simulink model "processor_128_channel_test"  (R2016b)
settings: Solver=VariableStepAuto  StartTime=0.0  StopTime=2^16/Fadc  RelTol=1e-3  EnableMultiTasking=on
PreLoadFcn:
  | setup
values from neighbouring files (symbols this model uses):
  Fadc = 614.4e6    (= 614400000)    [setup.m]
undefined symbols (not defined in the file or in its folder): etaTable, freqTable, gcbh, xlBlockLoadCallback
libraries: xbsIndex_r4 x44, CryoDetLibCMB x23, simulink x1
settings Model: Creator=Mitch  LastModifiedBy=mdewart
settings OptimizationCC: LifeSpan=inf
settings DebuggingCC: SFUnexpectedBacktrackingDiag=warning  SFNoUnconditionalDefaultTransitionDiag=warning  SFExecutionAtInitializationDiag=none
settings GRTTargetCC: TargetLangStandard=C89/C90 (ANSI)  GeneratePreprocessorConditionals=Disable all
settings ConfigComp: CovMetricSettings=dw  CovHtmlReporting=on  CovSaveCumulativeToWorkspaceVar=on  CovSaveSingleToWorkspaceVar=on  CovExternalEMLEnable=off

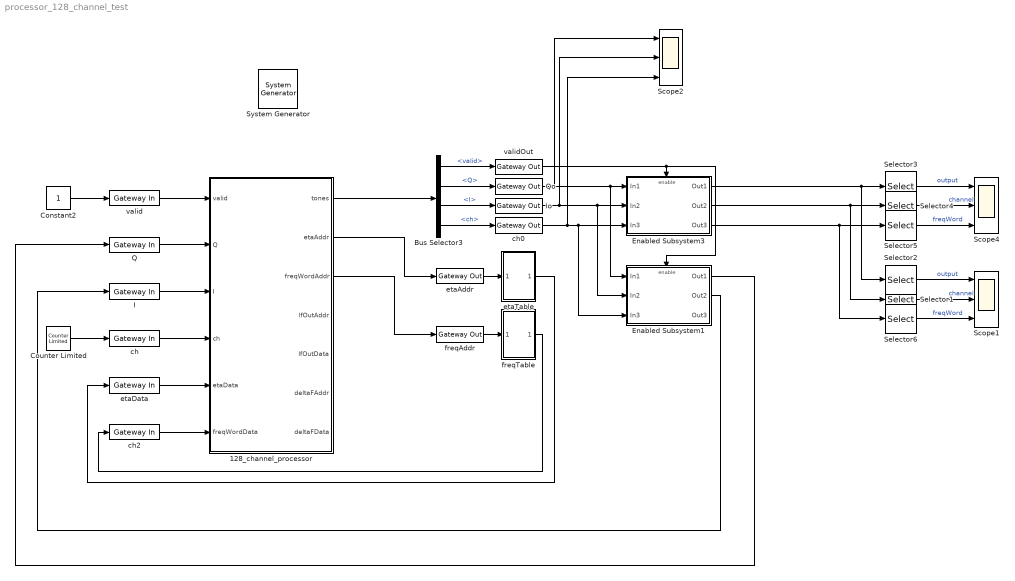
== system processor_128_channel_test ==
  " System Generator" : xbsIndex_r4/ System Generator  Tag=genX  xilinxfamily=kintexu  part=xcku040  speed=-2-e  package=ffva1156  synthesis_tool=Vivado  clock_wrapper=Clock Enables  directory=./netlist  proj_type=Vivado  Synth_file=Vivado Synthesis Defaults  Impl_file=Vivado Implementation Defaults  testbench=off  simulink_period=2/Fadc  sysclk_period=2e9/Fadc  dcm_input_clock_period=10  incr_netlist=off  trim_vbits=Everywhere in SubSystem  dbl_ovrd=According to Block Masks  core_generation=According to Block Masks  run_coregen=off  deprecated_control=off  eval_field=0  block_type=sysgen
  128_channel_processor : Subsystem  AncestorBlock=CryoDetLibCMB/128_channel_processor
  Bus Selector3 : BusSelector  OutputSignals=valid,Q,I,ch
  Constant2 : Constant  SampleTime=2/Fadc
  Counter Limited : simulink/Sources/Counter Limited  uplimit=7  tsamp=2/Fadc
  Enabled Subsystem1 : Subsystem  TreatAsAtomicUnit=on
  Enabled Subsystem3 : Subsystem  TreatAsAtomicUnit=on
  I : xbsIndex_r4/Gateway In  gui_display_data_type=Fixed-point  arith_type="Signed  (2's comp)"  n_bits=18  bin_pt=16  preci_type=Single  exp_width=8  frac_width=24  rows=1  columns=1  quantization="Round  (unbiased: +/- Inf)"  overflow=Saturate  period=2/Fadc  UseAsADC=off  ADCChannel='1'  interface=None  automatic_assignment=on  address_offset=hex2dec('00')  intf_name=''  intf_description=''  default_value=0  timing_constraint=None  locs_specified=off  LOCs={}  io_standard={}  inherit_from_input=off  hdl_port=on  dbl_ovrd=off  block_type=gatewayin
  Io : xbsIndex_r4/Gateway Out  inherit_from_input=off  hdl_port=on  rows=1  columns=1  UseAsDAC=off  DACChannel='1'  interface=None  automatic_assignment=on  address_offset=hex2dec('00')  intf_name=''  intf_description=''  timing_constraint=None  locs_specified=off  LOCs={}  io_standard={}  block_type=gatewayout
  Q : xbsIndex_r4/Gateway In  gui_display_data_type=Fixed-point  arith_type="Signed  (2's comp)"  n_bits=18  bin_pt=16  preci_type=Single  exp_width=8  frac_width=24  rows=1  columns=1  quantization="Round  (unbiased: +/- Inf)"  overflow=Saturate  period=2/Fadc  UseAsADC=off  ADCChannel='1'  interface=None  automatic_assignment=on  address_offset=hex2dec('00')  intf_name=''  intf_description=''  default_value=0  timing_constraint=None  locs_specified=off  LOCs={}  io_standard={}  inherit_from_input=off  hdl_port=on  dbl_ovrd=off  block_type=gatewayin
  Qo : xbsIndex_r4/Gateway Out  inherit_from_input=off  hdl_port=on  rows=1  columns=1  UseAsDAC=off  DACChannel='1'  interface=None  automatic_assignment=on  address_offset=hex2dec('00')  intf_name=''  intf_description=''  timing_constraint=None  locs_specified=off  LOCs={}  io_standard={}  block_type=gatewayout
  Scope1 : Scope  NumInputPorts=3
  Scope2 : Scope  NumInputPorts=3
  Scope4 : Scope  NumInputPorts=3
  Selector1 : Selector  InputPortWidth=8  IndexOptions=Index vector (dialog)  Indices=[7+1]  OutputSizes=1
  Selector2 : Selector  InputPortWidth=8  IndexOptions=Index vector (dialog)  Indices=[7+1]  OutputSizes=1
  Selector3 : Selector  InputPortWidth=8  IndexOptions=Index vector (dialog)  Indices=[1]  OutputSizes=1
  Selector4 : Selector  InputPortWidth=8  IndexOptions=Index vector (dialog)  Indices=[1]  OutputSizes=1
  Selector5 : Selector  InputPortWidth=8  IndexOptions=Index vector (dialog)  Indices=[1]  OutputSizes=1
  Selector6 : Selector  InputPortWidth=8  IndexOptions=Index vector (dialog)  Indices=[7+1]  OutputSizes=1
  ch : xbsIndex_r4/Gateway In  gui_display_data_type=Fixed-point  arith_type=Unsigned  n_bits=3  bin_pt=0  preci_type=Single  exp_width=8  frac_width=24  rows=1  columns=1  quantization="Round  (unbiased: +/- Inf)"  overflow=Saturate  period=2/Fadc  UseAsADC=off  ADCChannel='1'  interface=None  automatic_assignment=on  address_offset=hex2dec('00')  intf_name=''  intf_description=''  default_value=0  timing_constraint=None  locs_specified=off  LOCs={}  io_standard={}  inherit_from_input=off  hdl_port=on  dbl_ovrd=off  block_type=gatewayin
  ch0 : xbsIndex_r4/Gateway Out  inherit_from_input=off  hdl_port=on  rows=1  columns=1  UseAsDAC=off  DACChannel='1'  interface=None  automatic_assignment=on  address_offset=hex2dec('00')  intf_name=''  intf_description=''  timing_constraint=None  locs_specified=off  LOCs={}  io_standard={}  block_type=gatewayout
  ch2 : xbsIndex_r4/Gateway In  gui_display_data_type=Fixed-point  arith_type=Unsigned  n_bits=32  bin_pt=0  preci_type=Single  exp_width=8  frac_width=24  rows=1  columns=1  quantization="Round  (unbiased: +/- Inf)"  overflow=Saturate  period=2/Fadc  UseAsADC=off  ADCChannel='1'  interface=None  automatic_assignment=on  address_offset=hex2dec('00')  intf_name=''  intf_description=''  default_value=0  timing_constraint=None  locs_specified=off  LOCs={}  io_standard={}  inherit_from_input=off  hdl_port=on  dbl_ovrd=off  block_type=gatewayin
  etaAddr : xbsIndex_r4/Gateway Out  inherit_from_input=on  hdl_port=on  rows=1  columns=1  UseAsDAC=off  DACChannel='1'  interface=None  automatic_assignment=on  address_offset=hex2dec('00')  intf_name=''  intf_description=''  timing_constraint=None  locs_specified=off  LOCs={}  io_standard={}  block_type=gatewayout
  etaData : xbsIndex_r4/Gateway In  gui_display_data_type=Fixed-point  arith_type=Unsigned  n_bits=32  bin_pt=0  preci_type=Single  exp_width=8  frac_width=24  rows=1  columns=1  quantization="Round  (unbiased: +/- Inf)"  overflow=Saturate  period=2/Fadc  UseAsADC=off  ADCChannel='1'  interface=None  automatic_assignment=on  address_offset=hex2dec('00')  intf_name=''  intf_description=''  default_value=0  timing_constraint=None  locs_specified=off  LOCs={}  io_standard={}  inherit_from_input=off  hdl_port=on  dbl_ovrd=off  block_type=gatewayin
  etaTable : Subsystem
  freqAddr : xbsIndex_r4/Gateway Out  inherit_from_input=on  hdl_port=on  rows=1  columns=1  UseAsDAC=off  DACChannel='1'  interface=None  automatic_assignment=on  address_offset=hex2dec('00')  intf_name=''  intf_description=''  timing_constraint=None  locs_specified=off  LOCs={}  io_standard={}  block_type=gatewayout
  freqTable : Subsystem
  valid : xbsIndex_r4/Gateway In  gui_display_data_type=Boolean  arith_type=Boolean  n_bits=18  bin_pt=15  preci_type=Single  exp_width=8  frac_width=24  rows=1  columns=1  quantization="Round  (unbiased: +/- Inf)"  overflow=Saturate  period=2/Fadc  UseAsADC=off  ADCChannel='1'  interface=None  automatic_assignment=on  address_offset=hex2dec('00')  intf_name=''  intf_description=''  default_value=0  timing_constraint=None  locs_specified=off  LOCs={}  io_standard={}  inherit_from_input=off  hdl_port=on  dbl_ovrd=off  block_type=gatewayin
  validOut : xbsIndex_r4/Gateway Out  inherit_from_input=off  hdl_port=on  rows=1  columns=1  UseAsDAC=off  DACChannel='1'  interface=None  automatic_assignment=on  address_offset=hex2dec('00')  intf_name=''  intf_description=''  timing_constraint=None  locs_specified=off  LOCs={}  io_standard={}  block_type=gatewayout
  wires:
  Constant2/1 -> valid/1
  ch/1 -> 128_channel_processor/4(ch)
  valid/1 -> 128_channel_processor/1(valid)
  Bus Selector3/2 -> Qo/1  "<Q>"
  Bus Selector3/3 -> Io/1  "<I>"
  Bus Selector3/1 -> validOut/1  "<valid>"
  Bus Selector3/4 -> ch0/1  "<ch>"
  Selector3/1 -> Scope4/1  "output"
  Selector5/1 -> Scope4/3  "freqWord"
  Selector4/1 -> Scope4/2  "channel"
  Selector2/1 -> Scope1/1  "output"
  Selector6/1 -> Scope1/3  "freqWord"
  Selector1/1 -> Scope1/2  "channel"
  Q/1 -> 128_channel_processor/2(Q)
  Counter Limited/1 -> ch/1
  etaData/1 -> 128_channel_processor/5(etaData)
  ch2/1 -> 128_channel_processor/6(freqWordData)
  128_channel_processor/1(tones) -> Bus Selector3/1
  validOut/1 -> Enabled Subsystem1/Enable, Enabled Subsystem3/Enable
  ch0/1 -> Scope2/3, Enabled Subsystem1/3(In3), Enabled Subsystem3/3(In3)
  Io/1 -> Scope2/2, Enabled Subsystem1/2(In2), Enabled Subsystem3/2(In2)
  I/1 -> 128_channel_processor/3(I)
  Enabled Subsystem3/2(Out2) -> Selector1/1, Selector4/1
  128_channel_processor/2(etaAddr) -> etaAddr/1
  128_channel_processor/3(freqWordAddr) -> freqAddr/1
  Enabled Subsystem3/3(Out3) -> Selector6/1, Selector5/1
  Enabled Subsystem3/1(Out1) -> Selector2/1, Selector3/1
  etaAddr/1 -> etaTable/1(In1)
  freqAddr/1 -> freqTable/1(In1)
  freqTable/1(Out1) -> ch2/1
  etaTable/1(Out1) -> etaData/1
  Qo/1 -> Scope2/1, Enabled Subsystem1/1(In1), Enabled Subsystem3/1(In1)
  Enabled Subsystem1/1(Out1) -> Q/1
  Enabled Subsystem1/2(Out2) -> I/1

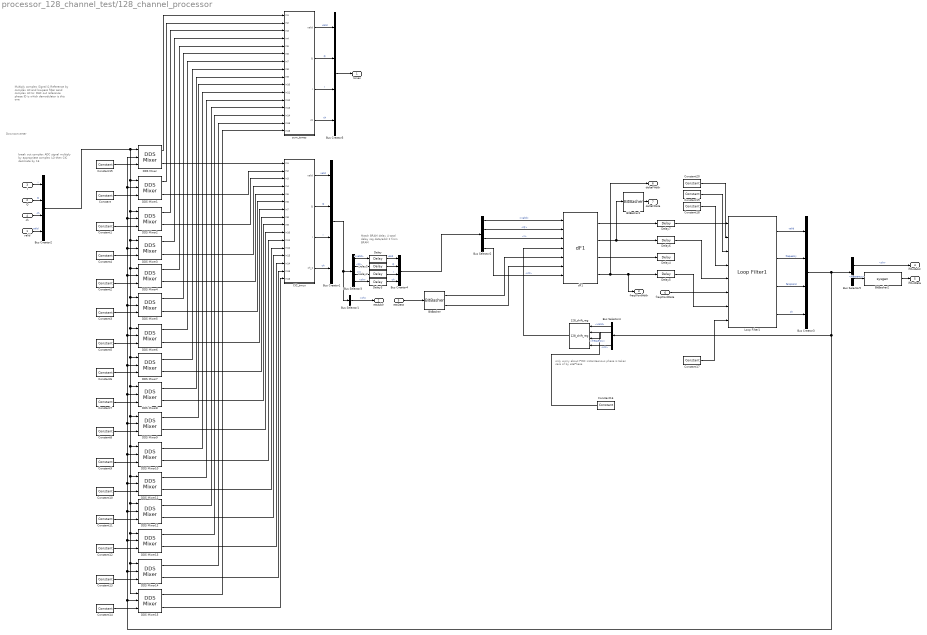
== system processor_128_channel_test/128_channel_processor ==
  note: Downconverter
  note: Multiply complex Signal & Reference
      | by complex LO and lowpass filter
      | send complex LO to:
      | 	DAC out
      | 	reference phase
      | ID is which demodulator is this one
  note: break out complex ADC signal
      | multiply by appropriate complex LO
      | then CIC decimate by 16
  note: Match BRAM delay
      | 4 total delay
      |    reg data/addr
      |    2 from BRAM
  note: only worry about PINC
      | instantaenous phase is taken care of by etaPhase
  valid : Inport
  Q : Inport  Port=2
  I : Inport  Port=3
  ch : Inport  Port=4
  etaData : Inport  Port=5
  freqWordData : Inport  Port=6
  128_shift_reg : CryoDetLibCMB/128_shift_reg
  BitBasher : xbsIndex_r4/BitBasher  bitexpr=|  display_expr=off  sr_1=etaPhase  arith_type1="Signed  (2's comp)"  bin_pt1=15  sr_2=etaMag  arith_type2="Signed  (2's comp)"  bin_pt2=10  sr_3=3  arith_type3=Unsigned  bin_pt3=0  sr_4=4  arith_type4=Unsigned  bin_pt4=0  dbl_ovrd=off  block_type=bitbasher
      | etaPhase = {in[31:16]}
      | etaMag = {in[15:0]}
  BitBasher1 : xbsIndex_r4/BitBasher  bitexpr=deltaF = {in[31:0]}  display_expr=off  sr_1=deltaF  arith_type1="Signed  (2's comp)"  bin_pt1=15  sr_2=etaMag  arith_type2="Signed  (2's comp)"  bin_pt2=10  sr_3=3  arith_type3=Unsigned  bin_pt3=0  sr_4=4  arith_type4=Unsigned  bin_pt4=0  dbl_ovrd=off  block_type=bitbasher
  BitBasher2 : S-Function  LoadFcn=xlBlockLoadCallback(gcbh);  FunctionName=sysgen  Parameters=ptable_  SFunctionDeploymentMode=off  EnableBusSupport=off  mask(Xilinx BitBasher Block){infoedit=Allows extraction, concatenation and augmentation of bits, bitexpr=loopFilterOut = {8'b0,in}, display_expr_sgadvanced=, display_expr=off, sr_1=loopFilterOut, arith_type1_sgadvanced=, arith_type1=Unsigned, bin_pt1=0, sr_2=etaMag, arith_type2_sgadvanced=, arith_type2=Signed  (2's comp), bin_pt2=10, sr_3=3, arith_type3_sgadvanced=, arith_type3=Unsigned, bin_pt3=0, sr_4=4, arith_type4_sgadvanced=, arith_type4=Unsigned, bin_pt4=0, dbl_ovrd=off, has_advanced_control=0, sggui_pos=20,45,368,336, block_type=bitbasher, block_version=, sg_icon_stat=120,42,1,1,white,blue,0,fb2ee5c8,right,,[ ],[ ], sg_mask_display=|, sg_list_contents=, sg_blockgui_xml=}
      mask sg_mask_display=|
      | fprintf('','COMMENT: begin icon graphics');
      | patch([0 120 120 0 0 ],[0 0 42 42 0 ],[0.77 0.82 0.91 ]);
      | plot([0 120 120 0 0 ],[0 0 42 42 0 ]);
      | patch([46.65 55.32 61.32 67.32 73.32 61.32 52.65 46.65 ],[27.66 27.66 33.66 27.66 33.66 33.66 33.66 27.66 ],[1 1 1 ]);
      | patch([52.65 61.32 55.32 46.65 52.65 ],[21.66 21.66 27.66 27.66 21.66 ],[0.931 0.946 0.973 ]);
      | patch([46.65 55.32 61.32 52.65 46.65 ],[15.66 15.66 21.66 21.66 15.66 ],[1 1 1 ]);
      | patch([52.65 73.32 67.32 61.32 55.32 46.65 52.65 ],[9.66 9.66 15.66 9.66 15.66 15.66 9.66 ],[0.931 0.946 0.973 ]);
      | fprintf('','COMMENT: end icon graphics');
      | fprintf('','COMMENT: begin icon text');
      | color('black');port_label('input',1,'in');
      | color('black');port_label('output',1,'loopFilterOut');
      | fprintf('','COMMENT: end icon text');
      mask prompts: infoedit ""; bitexpr "BitBasher Expression"; display_expr_sgadvanced ""; display_expr "Display expression on the block icon"; sr_1 ""; arith_type1_sgadvanced ""; arith_type1 ""; bin_pt1 ""; sr_2 ""; arith_type2_sgadvanced ""; arith_type2 ""; bin_pt2 ""; sr_3 ""; arith_type3_sgadvanced ""; arith_type3 ""; bin_pt3 ""; sr_4 ""; arith_type4_sgadvanced ""; arith_type4 ""; bin_pt4 ""; dbl_ovrd ""; has_advanced_control ""; sggui_pos ""; block_type ""; block_version ""; sg_icon_stat ""; sg_mask_display ""; sg_list_contents ""; sg_blockgui_xml ""
      mask help: Allows extraction, concatenation and augmentation of bits
      mask init:
      | try
      |   tmp_gcb = gcb;
      |   tmp_gcbh = gcbh;
      |   if (strcmp('SysGenIndex',get_param(bdroot(tmp_gcbh),'tag')) && ~isempty(regexp(bdroot(tmp_gcb), '^xbs', 'once')))
      |     return;
      |   end;
      |   xlMungeMaskParams;
      |   block_config = 'sysgen:BitBasher_config';
      | 
      |   block_type='bitbasher';
      | 
      |   serialized_declarations = '{''arith_type1''=>''Int'',''arith_type2''=>''Int'',''arith_type3''=>''Int'',''arith_type4''=>''Int'',''bin_pt1''=>''Int'',''bin_pt2''=>''Int'',''bin_pt3''=>''Int'',''bin_pt4''=>''Int'',''bitexpr''=>''String'',''chksum''=>''String'',''dbl_ovrd''=>''String'',''display_expr''=>''Int'',''sim_engine''=>''Int'',''sysgen_root''=>''String'',''xinports''=>''DoubleVector'',''xoutports''=>''DoubleVector'',''block_type''=>''String''}';
      |   xlbitbasher_init();
      |   ptable_ = xlblockprep(get_param(tmp_gcb, 'MaskWSVariables'));
      |   try
      |     xlBlockMoveCallback(tmp_gcbh);
      |   catch 
      |      clear global xl_updateicon_recursion_guard;
      |   end;
      | catch
      |   global dbgsysgen;
      |   if(~isempty(dbgsysgen) && dbgsysgen)
      |     e = regexprep(lasterr, '\n', '\nError: ');
      |     disp(['Error: While running MaskInit code on block ' tmp_gcb ': ' e]);
      |     error(e);
      |   end
      | end
      settings: CopyFcn=xlBlockMoveCallback(gcbh);  DeleteFcn=xlDestroyGui(gcbh);  ModelCloseFcn=xlDestroyGui(gcbh);  PreSaveFcn=xlBlockPreSaveCallback(gcbh);  PostSaveFcn=xlBlockPostSaveCallback(gcbh);  DestroyFcn=xlDestroyGui(gcbh);  OpenFcn=xlOpenGui(gcbh, 'bitbasher_gui.xml', @bitbasherenablement, @bitbasheraction)  CloseFcn=xlDestroyGui(gcbh);  MoveFcn=xlBlockMoveCallback(gcbh);
      mask Help: eval('');xlDoc('-book','sysgen','-topic','BitBasher');
      mask TypeOptions arith_type1: Unsigned | Signed  (2's comp)
      mask TypeOptions arith_type2: Unsigned | Signed  (2's comp)
      mask TypeOptions arith_type3: Unsigned | Signed  (2's comp)
      mask TypeOptions arith_type4: Unsigned | Signed  (2's comp)
      mask Display:
      | fprintf('','COMMENT: begin icon graphics');
      | patch([0 120 120 0 0 ],[0 0 42 42 0 ],[0.77 0.82 0.91 ]);
      | plot([0 120 120 0 0 ],[0 0 42 42 0 ]);
      | patch([46.65 55.32 61.32 67.32 73.32 61.32 52.65 46.65 ],[27.66 27.66 33.66 27.66 33.66 33.66 33.66 27.66 ],[1 1 1 ]);
      | patch([52.65 61.32 55.32 46.65 52.65 ],[21.66 21.66 27.66 27.66 21.66 ],[0.931 0.946 0.973 ]);
      | patch([46.65 55.32 61.32 52.65 46.65 ],[15.66 15.66 21.66 21.66 15.66 ],[1 1 1 ]);
      | patch([52.65 73.32 67.32 61.32 55.32 46.65 52.65 ],[9.66 9.66 15.66 9.66 15.66 15.66 9.66 ],[0.931 0.946 0.973 ]);
      | fprintf('','COMMENT: end icon graphics');
      | fprintf('','COMMENT: begin icon text');
      | color('black');port_label('input',1,'in');
      | color('black');port_label('output',1,'loopFilterOut');
      | fprintf('','COMMENT: end icon text');
  Bus Creator{1..5} (5 alike) : BusCreator  Inputs=4
  Bus Selector1 : BusSelector  OutputSignals=ch
  Bus Selector2 : BusSelector  OutputSignals=valid,Q,I,ch
  Bus Selector3 : BusSelector  OutputSignals=valid,Q,I,ch
  Bus Selector4 : BusSelector  OutputSignals=valid,frequency,ferqWord,ch
  Bus Selector5 : BusSelector  OutputSignals=ch,frequency
  CIC_tmux : Subsystem
  Constant : xbsIndex_r4/Constant  const=1  gui_display_data_type=Fixed-point  arith_type=Unsigned  n_bits=4  bin_pt=0  preci_type=Single  exp_width=8  frac_width=24  explicit_period=off  period=1  equ=P=C  opselect=C  inp2=PCIN>>17  opr=+  inp1=P  carry=CIN  dbl_ovrd=off  block_type=constant
  Constant1 : xbsIndex_r4/Constant  const=2  gui_display_data_type=Fixed-point  arith_type=Unsigned  n_bits=4  bin_pt=0  preci_type=Single  exp_width=8  frac_width=24  explicit_period=off  period=1  equ=P=C  opselect=C  inp2=PCIN>>17  opr=+  inp1=P  carry=CIN  dbl_ovrd=off  block_type=constant
  Constant10 : xbsIndex_r4/Constant  const=11  gui_display_data_type=Fixed-point  arith_type=Unsigned  n_bits=4  bin_pt=0  preci_type=Single  exp_width=8  frac_width=24  explicit_period=off  period=1  equ=P=C  opselect=C  inp2=PCIN>>17  opr=+  inp1=P  carry=CIN  dbl_ovrd=off  block_type=constant
  Constant11 : xbsIndex_r4/Constant  const=12  gui_display_data_type=Fixed-point  arith_type=Unsigned  n_bits=4  bin_pt=0  preci_type=Single  exp_width=8  frac_width=24  explicit_period=off  period=1  equ=P=C  opselect=C  inp2=PCIN>>17  opr=+  inp1=P  carry=CIN  dbl_ovrd=off  block_type=constant
  Constant12 : xbsIndex_r4/Constant  const=13  gui_display_data_type=Fixed-point  arith_type=Unsigned  n_bits=4  bin_pt=0  preci_type=Single  exp_width=8  frac_width=24  explicit_period=off  period=1  equ=P=C  opselect=C  inp2=PCIN>>17  opr=+  inp1=P  carry=CIN  dbl_ovrd=off  block_type=constant
  Constant13 : xbsIndex_r4/Constant  const=14  gui_display_data_type=Fixed-point  arith_type=Unsigned  n_bits=4  bin_pt=0  preci_type=Single  exp_width=8  frac_width=24  explicit_period=off  period=1  equ=P=C  opselect=C  inp2=PCIN>>17  opr=+  inp1=P  carry=CIN  dbl_ovrd=off  block_type=constant
  Constant14 : xbsIndex_r4/Constant  const=15  gui_display_data_type=Fixed-point  arith_type=Unsigned  n_bits=4  bin_pt=0  preci_type=Single  exp_width=8  frac_width=24  explicit_period=off  period=1  equ=P=C  opselect=C  inp2=PCIN>>17  opr=+  inp1=P  carry=CIN  dbl_ovrd=off  block_type=constant
  Constant15 : xbsIndex_r4/Constant  const=0  gui_display_data_type=Fixed-point  arith_type=Unsigned  n_bits=4  bin_pt=0  preci_type=Single  exp_width=8  frac_width=24  explicit_period=off  period=1  equ=P=C  opselect=C  inp2=PCIN>>17  opr=+  inp1=P  carry=CIN  dbl_ovrd=off  block_type=constant
  Constant16 : xbsIndex_r4/Constant  const=0  gui_display_data_type=Fixed-point  arith_type=Unsigned  n_bits=3  bin_pt=0  preci_type=Single  exp_width=8  frac_width=24  explicit_period=on  period=2/Fadc  equ=P=C  opselect=C  inp2=PCIN>>17  opr=+  inp1=P  carry=CIN  dbl_ovrd=off  block_type=constant
  Constant17 : xbsIndex_r4/Constant  const=0  gui_display_data_type=Fixed-point  arith_type=Unsigned  n_bits=3  bin_pt=0  preci_type=Single  exp_width=8  frac_width=24  explicit_period=on  period=2/Fadc  equ=P=C  opselect=C  inp2=PCIN>>17  opr=+  inp1=P  carry=CIN  dbl_ovrd=off  block_type=constant
  Constant18 : xbsIndex_r4/Constant  const=1  gui_display_data_type=Fixed-point  arith_type=Signed (2's comp)  n_bits=32  bin_pt=30  preci_type=Single  exp_width=8  frac_width=24  explicit_period=on  period=2/Fadc  equ=P=C  opselect=C  inp2=PCIN>>17  opr=+  inp1=P  carry=CIN  dbl_ovrd=off  block_type=constant
  Constant19 : xbsIndex_r4/Constant  const=1  gui_display_data_type=Fixed-point  arith_type=Signed (2's comp)  n_bits=17  bin_pt=14  preci_type=Single  exp_width=8  frac_width=24  explicit_period=on  period=2/Fadc  equ=P=C  opselect=C  inp2=PCIN>>17  opr=+  inp1=P  carry=CIN  dbl_ovrd=off  block_type=constant
  Constant2 : xbsIndex_r4/Constant  const=4  gui_display_data_type=Fixed-point  arith_type=Unsigned  n_bits=4  bin_pt=0  preci_type=Single  exp_width=8  frac_width=24  explicit_period=off  period=1  equ=P=C  opselect=C  inp2=PCIN>>17  opr=+  inp1=P  carry=CIN  dbl_ovrd=off  block_type=constant
  Constant20 : xbsIndex_r4/Constant  const=0  gui_display_data_type=Fixed-point  arith_type=Unsigned  n_bits=1  bin_pt=0  preci_type=Single  exp_width=8  frac_width=24  explicit_period=on  period=2/Fadc  equ=P=C  opselect=C  inp2=PCIN>>17  opr=+  inp1=P  carry=CIN  dbl_ovrd=off  block_type=constant
  Constant3 : xbsIndex_r4/Constant  const=5  gui_display_data_type=Fixed-point  arith_type=Unsigned  n_bits=4  bin_pt=0  preci_type=Single  exp_width=8  frac_width=24  explicit_period=off  period=1  equ=P=C  opselect=C  inp2=PCIN>>17  opr=+  inp1=P  carry=CIN  dbl_ovrd=off  block_type=constant
  Constant4 : xbsIndex_r4/Constant  const=3  gui_display_data_type=Fixed-point  arith_type=Unsigned  n_bits=4  bin_pt=0  preci_type=Single  exp_width=8  frac_width=24  explicit_period=off  period=1  equ=P=C  opselect=C  inp2=PCIN>>17  opr=+  inp1=P  carry=CIN  dbl_ovrd=off  block_type=constant
  Constant5 : xbsIndex_r4/Constant  const=6  gui_display_data_type=Fixed-point  arith_type=Unsigned  n_bits=4  bin_pt=0  preci_type=Single  exp_width=8  frac_width=24  explicit_period=off  period=1  equ=P=C  opselect=C  inp2=PCIN>>17  opr=+  inp1=P  carry=CIN  dbl_ovrd=off  block_type=constant
  Constant6 : xbsIndex_r4/Constant  const=7  gui_display_data_type=Fixed-point  arith_type=Unsigned  n_bits=4  bin_pt=0  preci_type=Single  exp_width=8  frac_width=24  explicit_period=off  period=1  equ=P=C  opselect=C  inp2=PCIN>>17  opr=+  inp1=P  carry=CIN  dbl_ovrd=off  block_type=constant
  Constant7 : xbsIndex_r4/Constant  const=8  gui_display_data_type=Fixed-point  arith_type=Unsigned  n_bits=4  bin_pt=0  preci_type=Single  exp_width=8  frac_width=24  explicit_period=off  period=1  equ=P=C  opselect=C  inp2=PCIN>>17  opr=+  inp1=P  carry=CIN  dbl_ovrd=off  block_type=constant
  Constant8 : xbsIndex_r4/Constant  const=9  gui_display_data_type=Fixed-point  arith_type=Unsigned  n_bits=4  bin_pt=0  preci_type=Single  exp_width=8  frac_width=24  explicit_period=off  period=1  equ=P=C  opselect=C  inp2=PCIN>>17  opr=+  inp1=P  carry=CIN  dbl_ovrd=off  block_type=constant
  Constant9 : xbsIndex_r4/Constant  const=10  gui_display_data_type=Fixed-point  arith_type=Unsigned  n_bits=4  bin_pt=0  preci_type=Single  exp_width=8  frac_width=24  explicit_period=off  period=1  equ=P=C  opselect=C  inp2=PCIN>>17  opr=+  inp1=P  carry=CIN  dbl_ovrd=off  block_type=constant
  DDS Mixer{,1..15} (16 alike) : CryoDetLibCMB/DDS Mixer
  Delay{,1..7} (8 alike) : xbsIndex_r4/Delay  rst=off  infoeditControl=Selection of Reset will increase slice count due to use of real FFs and instead of SRLs  en=off  latency=4  reg_retiming=off  dbl_ovrd=off  block_type=delay
  Loop Filter1 : CryoDetLibCMB/Loop Filter1
  dF1 : CryoDetLibCMB/dF1
      link override Reinterpret: force_arith_type=on  arith_type=Unsigned  force_bin_pt=on  bin_pt=0
      link override Reinterpret1: force_arith_type=on  arith_type="Signed  (2's comp)"  force_bin_pt=on  bin_pt=10
      link override Reinterpret: infoedit="Changes signal type without altering the binary representation.   You can change the signal between signed and unsigned, and relocate the binary point.<br><br>Hardware notes: In hardware this block costs nothing.<br><br>Example:  Suppose the input is 6 bits wide, signed, with 2 fractional bits, and the output is forced to unsigned with 0 fractional bits.  Then an input of -2.0 (1110.00 in binary 2's complement) becomes an output of 56 (111000 in binary)."
      link override Reinterpret1: infoedit="Changes signal type without altering the binary representation.   You can change the signal between signed and unsigned, and relocate the binary point.<br><br>Hardware notes: In hardware this block costs nothing.<br><br>Example:  Suppose the input is 6 bits wide, signed, with 2 fractional bits, and the output is forced to unsigned with 0 fractional bits.  Then an input of -2.0 (1110.00 in binary 2's complement) becomes an output of 56 (111000 in binary)."
  sum_tones : Subsystem
  tones : Outport
  etaAddr : Outport  Port=2
  freqWordAddr : Outport  Port=3
  lfOutAddr : Outport  Port=4
  lfOutData : Outport  Port=5
  deltaFAddr : Outport  Port=6
  deltaFData : Outport  Port=7
  wires:
  Bus Selector5/1 -> lfOutAddr/1  "<ch>"
  Bus Selector5/2 -> BitBasher2/1  "<frequency>"
  BitBasher2/1 -> lfOutData/1
  Bus Selector4/1 -> 128_shift_reg/1  "<valid>"
  Bus Selector4/2 -> 128_shift_reg/3  "<frequency>"
  Bus Selector4/4 -> 128_shift_reg/4  "<ch>"
  Loop Filter1/4 -> Bus Creator3/4  "ch"
  Loop Filter1/3 -> Bus Creator3/3  "ferqWord"
  Loop Filter1/2 -> Bus Creator3/2  "frequency"
  Loop Filter1/1 -> Bus Creator3/1  "valid"
  Delay5/1 -> Loop Filter1/7
  freqWordData/1 -> Loop Filter1/6
  Delay6/1 -> Loop Filter1/5
  Delay7/1 -> Loop Filter1/1
  dF1/1 -> Delay7/1
  dF1/2 -> Delay6/1, BitBasher1/1
  128_shift_reg/2 -> dF1/4
  Bus Selector2/4 -> dF1/7  "<ch>"
  BitBasher/2 -> dF1/6
  BitBasher/1 -> dF1/5
  Bus Selector2/3 -> dF1/3  "<I>"
  Bus Selector2/2 -> dF1/2  "<Q>"
  Bus Selector2/1 -> dF1/1  "<valid>"
  Bus Creator5/1 -> tones/1
  sum_tones/1(valid) -> Bus Creator5/1  "valid"
  sum_tones/4(ch) -> Bus Creator5/4  "ch"
  sum_tones/2(Q) -> Bus Creator5/2  "Q"
  sum_tones/3(I) -> Bus Creator5/3  "I"
  Bus Selector3/4 -> Delay3/1  "<ch>"
  Bus Selector3/3 -> Delay2/1  "<I>"
  Bus Selector3/2 -> Delay1/1  "<Q>"
  Bus Selector3/1 -> Delay/1  "<valid>"
  CIC_tmux/4(ch_o) -> Bus Creator1/4  "ch"
  CIC_tmux/3(I) -> Bus Creator1/3  "I"
  CIC_tmux/2(Q) -> Bus Creator1/2  "Q"
  CIC_tmux/1(valid) -> Bus Creator1/1  "valid"
  dF1/3 -> Delay4/1
  dF1/4 -> deltaFAddr/1, Delay5/1, freqWordAddr/1
  BitBasher1/1 -> deltaFData/1
  Bus Creator4/1 -> Bus Selector2/1
  etaData/1 -> BitBasher/1
  Delay3/1 -> Bus Creator4/4  "ch"
  Delay2/1 -> Bus Creator4/3  "I"
  Delay1/1 -> Bus Creator4/2  "Q"
  Delay/1 -> Bus Creator4/1  "valid"
  Bus Selector1/1 -> etaAddr/1  "<ch>"
  Bus Creator1/1 -> Bus Selector1/1, Bus Selector3/1
  valid/1 -> Bus Creator2/4  "valid"
  ch/1 -> Bus Creator2/3  "ch"
  Q/1 -> Bus Creator2/2  "Q"
  I/1 -> Bus Creator2/1  "I"
  DDS Mixer15/1 -> sum_tones/16(In16)
  DDS Mixer14/1 -> sum_tones/15(In15)
  DDS Mixer13/1 -> sum_tones/14(In14)
  DDS Mixer12/1 -> sum_tones/13(In13)
  DDS Mixer11/1 -> sum_tones/12(In12)
  DDS Mixer10/1 -> sum_tones/11(In11)
  DDS Mixer9/1 -> sum_tones/10(In10)
  DDS Mixer8/1 -> sum_tones/9(In9)
  DDS Mixer7/1 -> sum_tones/8(In8)
  DDS Mixer6/1 -> sum_tones/7(In7)
  DDS Mixer5/1 -> sum_tones/6(In6)
  DDS Mixer4/1 -> sum_tones/5(In5)
  DDS Mixer3/1 -> sum_tones/4(In4)
  DDS Mixer2/1 -> sum_tones/3(In3)
  DDS Mixer1/1 -> sum_tones/2(In2)
  DDS Mixer/1 -> sum_tones/1(In1)
  Constant15/1 -> DDS Mixer/3
  Constant5/1 -> DDS Mixer6/3
  Constant6/1 -> DDS Mixer7/3
  Constant7/1 -> DDS Mixer8/3
  Constant8/1 -> DDS Mixer9/3
  Constant9/1 -> DDS Mixer10/3
  Constant10/1 -> DDS Mixer11/3
  Constant11/1 -> DDS Mixer12/3
  Constant12/1 -> DDS Mixer13/3
  Constant13/1 -> DDS Mixer14/3
  Constant14/1 -> DDS Mixer15/3
  Constant4/1 -> DDS Mixer3/3
  Constant3/1 -> DDS Mixer5/3
  Constant2/1 -> DDS Mixer4/3
  Constant1/1 -> DDS Mixer2/3
  Constant/1 -> DDS Mixer1/3
  Bus Creator3/1 -> Bus Selector4/1, DDS Mixer15/2, DDS Mixer14/2, DDS Mixer13/2, DDS Mixer12/2, DDS Mixer11/2, DDS Mixer10/2, DDS Mixer9/2, DDS Mixer8/2, DDS Mixer7/2, DDS Mixer6/2, DDS Mixer5/2, DDS Mixer4/2, DDS Mixer3/2, DDS Mixer2/2, DDS Mixer1/2, DDS Mixer/2, Bus Selector5/1
  Bus Creator2/1 -> DDS Mixer/1, DDS Mixer1/1, DDS Mixer8/1, DDS Mixer15/1, DDS Mixer14/1, DDS Mixer13/1, DDS Mixer12/1, DDS Mixer11/1, DDS Mixer10/1, DDS Mixer9/1, DDS Mixer7/1, DDS Mixer6/1, DDS Mixer5/1, DDS Mixer4/1, DDS Mixer3/1, DDS Mixer2/1
  DDS Mixer15/2 -> CIC_tmux/16(In16)
  DDS Mixer14/2 -> CIC_tmux/15(In15)
  DDS Mixer13/2 -> CIC_tmux/14(In14)
  DDS Mixer12/2 -> CIC_tmux/13(In13)
  DDS Mixer11/2 -> CIC_tmux/12(In12)
  DDS Mixer10/2 -> CIC_tmux/11(In11)
  DDS Mixer9/2 -> CIC_tmux/10(In10)
  DDS Mixer8/2 -> CIC_tmux/9(In9)
  DDS Mixer7/2 -> CIC_tmux/8(In8)
  DDS Mixer6/2 -> CIC_tmux/7(In7)
  DDS Mixer5/2 -> CIC_tmux/6(In6)
  DDS Mixer4/2 -> CIC_tmux/5(In5)
  DDS Mixer3/2 -> CIC_tmux/4(In4)
  DDS Mixer2/2 -> CIC_tmux/3(In3)
  DDS Mixer1/2 -> CIC_tmux/2(In2)
  DDS Mixer/2 -> CIC_tmux/1(In1)
  Constant16/1 -> 128_shift_reg/2
  Constant17/1 -> Loop Filter1/8
  Constant18/1 -> Loop Filter1/4
  Constant19/1 -> Loop Filter1/3
  Constant20/1 -> Loop Filter1/2

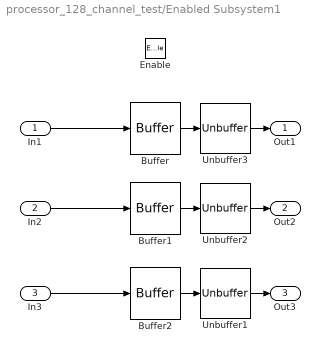
== system processor_128_channel_test/Enabled Subsystem1 ==
  In1 : Inport
  In2 : Inport  Port=2
  In3 : Inport  Port=3
  Enable : EnablePort
  Buffer : Buffer  N=8  TreatMby1Signals=One channel  OutputFrames=off
  Buffer1 : Buffer  N=8  TreatMby1Signals=One channel  OutputFrames=off
  Buffer2 : Buffer  N=8  TreatMby1Signals=One channel  OutputFrames=off
  Unbuffer1 : Unbuffer  SampleBasedProcessing=Same as frame based
  Unbuffer2 : Unbuffer  SampleBasedProcessing=Same as frame based
  Unbuffer3 : Unbuffer  SampleBasedProcessing=Same as frame based
  Out1 : Outport
  Out2 : Outport  Port=2
  Out3 : Outport  Port=3
  wires:
  In3/1 -> Buffer2/1
  Buffer1/1 -> Unbuffer2/1
  In2/1 -> Buffer1/1
  Buffer/1 -> Unbuffer3/1
  In1/1 -> Buffer/1
  Buffer2/1 -> Unbuffer1/1
  Unbuffer1/1 -> Out3/1
  Unbuffer2/1 -> Out2/1
  Unbuffer3/1 -> Out1/1

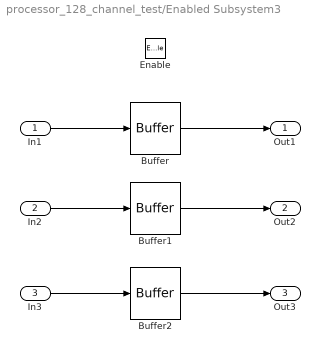
== system processor_128_channel_test/Enabled Subsystem3 ==
  In1 : Inport
  In2 : Inport  Port=2
  In3 : Inport  Port=3
  Enable : EnablePort
  Buffer : Buffer  N=8  TreatMby1Signals=One channel  OutputFrames=off
  Buffer1 : Buffer  N=8  TreatMby1Signals=One channel  OutputFrames=off
  Buffer2 : Buffer  N=8  TreatMby1Signals=One channel  OutputFrames=off
  Out1 : Outport
  Out2 : Outport  Port=2
  Out3 : Outport  Port=3
  wires:
  In1/1 -> Buffer/1
  Buffer/1 -> Out1/1
  In2/1 -> Buffer1/1
  Buffer1/1 -> Out2/1
  In3/1 -> Buffer2/1
  Buffer2/1 -> Out3/1

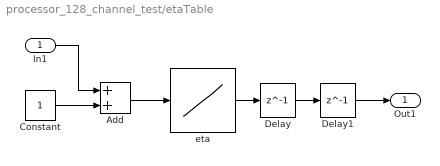
== system processor_128_channel_test/etaTable ==
  In1 : Inport
  Add : Sum
  Constant : Constant
  Delay : Delay  DelayLength=1  InitialCondition=0
  Delay1 : Delay  DelayLength=1  InitialCondition=0
  eta : Lookup_n-D  NumberOfTableDimensions=1  BreakpointsSpecification=Even spacing  BreakpointsForDimension1=[-5:5]  Table=etaTable  TableDataTypeStr=uint32  InterpMethod=Nearest  InternalRulePriority=Speed  OutDataTypeStr=uint32  RndMeth=Simplest  InputSameDT=on
  Out1 : Outport
  wires:
  Delay/1 -> Delay1/1
  Delay1/1 -> Out1/1
  eta/1 -> Delay/1
  Constant/1 -> Add/2
  Add/1 -> eta/1
  In1/1 -> Add/1

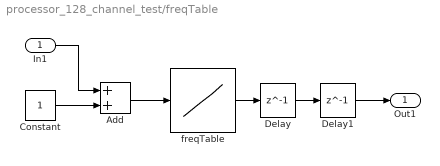
== system processor_128_channel_test/freqTable ==
  In1 : Inport
  Add : Sum
  Constant : Constant
  Delay : Delay  DelayLength=1  InitialCondition=0
  Delay1 : Delay  DelayLength=1  InitialCondition=0
  freqTable : Lookup_n-D  NumberOfTableDimensions=1  BreakpointsSpecification=Even spacing  BreakpointsForDimension1=[-5:5]  Table=freqTable  TableDataTypeStr=uint32  InterpMethod=Nearest  InternalRulePriority=Speed  OutDataTypeStr=uint32  RndMeth=Simplest  InputSameDT=on
  Out1 : Outport
  wires:
  In1/1 -> Add/1
  Add/1 -> freqTable/1
  Constant/1 -> Add/2
  freqTable/1 -> Delay/1
  Delay1/1 -> Out1/1
  Delay/1 -> Delay1/1

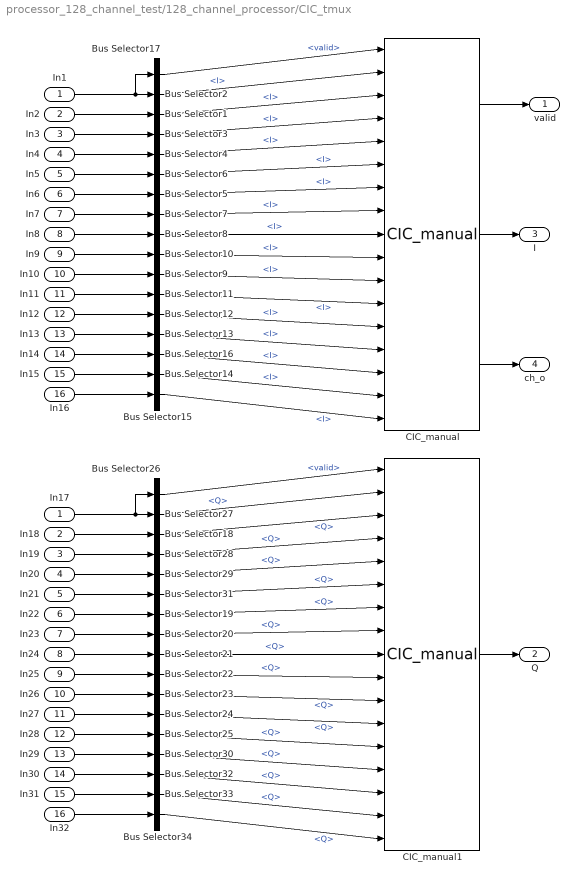
== system processor_128_channel_test/128_channel_processor/CIC_tmux ==
  In1 : Inport
  In2 : Inport  Port=2
  In3 : Inport  Port=3
  In4 : Inport  Port=4
  In5 : Inport  Port=5
  In6 : Inport  Port=6
  In7 : Inport  Port=7
  In8 : Inport  Port=8
  In9 : Inport  Port=9
  In10 : Inport  Port=10
  In11 : Inport  Port=11
  In12 : Inport  Port=12
  In13 : Inport  Port=13
  In14 : Inport  Port=14
  In15 : Inport  Port=15
  In16 : Inport  Port=16
  Bus Selector{1..16} (16 alike) : BusSelector  OutputSignals=I
  Bus Selector17 : BusSelector  OutputSignals=valid
  Bus Selector{18..25,27..34} (16 alike) : BusSelector  OutputSignals=Q
  Bus Selector26 : BusSelector  OutputSignals=valid
  CIC_manual : CryoDetLibCMB/CIC_manual  n_bit=18  b_pt=0
  CIC_manual1 : CryoDetLibCMB/CIC_manual  n_bit=18  b_pt=0
      link override RST: const=0  gui_display_data_type=Boolean  arith_type=Boolean  n_bits=16  bin_pt=14  preci_type=Single  exp_width=8  frac_width=24  explicit_period=on  period=2/Fadc  equ=P=C  opselect=C  inp2=PCIN>>17  opr=+  inp1=P  carry=CIN  dbl_ovrd=off
  In17 : InportShadow
  In18 : InportShadow  Port=2
  In19 : InportShadow  Port=3
  In20 : InportShadow  Port=4
  In21 : InportShadow  Port=5
  In22 : InportShadow  Port=6
  In23 : InportShadow  Port=7
  In24 : InportShadow  Port=8
  In25 : InportShadow  Port=9
  In26 : InportShadow  Port=10
  In27 : InportShadow  Port=11
  In28 : InportShadow  Port=12
  In29 : InportShadow  Port=13
  In30 : InportShadow  Port=14
  In31 : InportShadow  Port=15
  In32 : InportShadow  Port=16
  valid : Outport
  Q : Outport  Port=2
  I : Outport  Port=3
  ch_o : Outport  Port=4
  wires:
  CIC_manual1/2 -> Q/1
  CIC_manual/3 -> ch_o/1
  CIC_manual/1 -> valid/1
  CIC_manual/2 -> I/1
  Bus Selector34/1 -> CIC_manual1/17  "<Q>"
  Bus Selector33/1 -> CIC_manual1/16  "<Q>"
  Bus Selector32/1 -> CIC_manual1/15  "<Q>"
  Bus Selector31/1 -> CIC_manual1/6  "<Q>"
  Bus Selector30/1 -> CIC_manual1/14  "<Q>"
  Bus Selector29/1 -> CIC_manual1/5  "<Q>"
  Bus Selector28/1 -> CIC_manual1/4  "<Q>"
  Bus Selector27/1 -> CIC_manual1/2  "<Q>"
  Bus Selector26/1 -> CIC_manual1/1  "<valid>"
  Bus Selector25/1 -> CIC_manual1/13  "<Q>"
  Bus Selector24/1 -> CIC_manual1/12  "<Q>"
  Bus Selector23/1 -> CIC_manual1/11  "<Q>"
  Bus Selector22/1 -> CIC_manual1/10  "<Q>"
  Bus Selector21/1 -> CIC_manual1/9  "<Q>"
  Bus Selector20/1 -> CIC_manual1/8  "<Q>"
  Bus Selector19/1 -> CIC_manual1/7  "<Q>"
  Bus Selector18/1 -> CIC_manual1/3  "<Q>"
  Bus Selector9/1 -> CIC_manual/11  "<I>"
  Bus Selector8/1 -> CIC_manual/9  "<I>"
  Bus Selector7/1 -> CIC_manual/8  "<I>"
  Bus Selector6/1 -> CIC_manual/6  "<I>"
  Bus Selector5/1 -> CIC_manual/7  "<I>"
  Bus Selector4/1 -> CIC_manual/5  "<I>"
  Bus Selector3/1 -> CIC_manual/4  "<I>"
  Bus Selector2/1 -> CIC_manual/2  "<I>"
  Bus Selector17/1 -> CIC_manual/1  "<valid>"
  Bus Selector16/1 -> CIC_manual/15  "<I>"
  Bus Selector15/1 -> CIC_manual/17  "<I>"
  Bus Selector14/1 -> CIC_manual/16  "<I>"
  Bus Selector13/1 -> CIC_manual/14  "<I>"
  Bus Selector12/1 -> CIC_manual/13  "<I>"
  Bus Selector11/1 -> CIC_manual/12  "<I>"
  Bus Selector10/1 -> CIC_manual/10  "<I>"
  Bus Selector1/1 -> CIC_manual/3  "<I>"
  In32/1 -> Bus Selector34/1
  In31/1 -> Bus Selector33/1
  In30/1 -> Bus Selector32/1
  In29/1 -> Bus Selector30/1
  In28/1 -> Bus Selector25/1
  In27/1 -> Bus Selector24/1
  In26/1 -> Bus Selector23/1
  In25/1 -> Bus Selector22/1
  In24/1 -> Bus Selector21/1
  In23/1 -> Bus Selector20/1
  In22/1 -> Bus Selector19/1
  In21/1 -> Bus Selector31/1
  In20/1 -> Bus Selector29/1
  In19/1 -> Bus Selector28/1
  In18/1 -> Bus Selector18/1
  In17/1 -> Bus Selector26/1, Bus Selector27/1
  In16/1 -> Bus Selector15/1
  In15/1 -> Bus Selector14/1
  In14/1 -> Bus Selector16/1
  In13/1 -> Bus Selector13/1
  In12/1 -> Bus Selector12/1
  In11/1 -> Bus Selector11/1
  In10/1 -> Bus Selector9/1
  In9/1 -> Bus Selector10/1
  In8/1 -> Bus Selector8/1
  In7/1 -> Bus Selector7/1
  In6/1 -> Bus Selector5/1
  In5/1 -> Bus Selector6/1
  In4/1 -> Bus Selector4/1
  In3/1 -> Bus Selector3/1
  In2/1 -> Bus Selector1/1
  In1/1 -> Bus Selector2/1, Bus Selector17/1

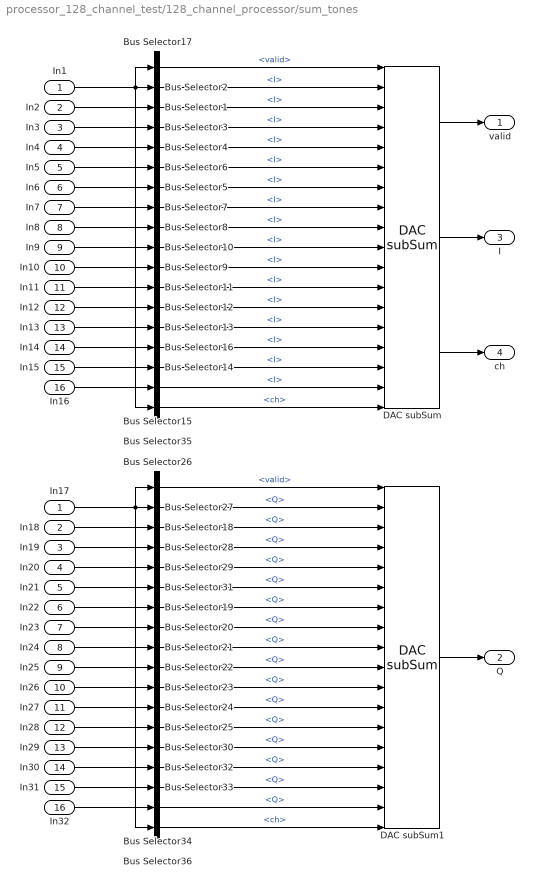
== system processor_128_channel_test/128_channel_processor/sum_tones ==
  In1 : Inport
  In2 : Inport  Port=2
  In3 : Inport  Port=3
  In4 : Inport  Port=4
  In5 : Inport  Port=5
  In6 : Inport  Port=6
  In7 : Inport  Port=7
  In8 : Inport  Port=8
  In9 : Inport  Port=9
  In10 : Inport  Port=10
  In11 : Inport  Port=11
  In12 : Inport  Port=12
  In13 : Inport  Port=13
  In14 : Inport  Port=14
  In15 : Inport  Port=15
  In16 : Inport  Port=16
  Bus Selector{1..16} (16 alike) : BusSelector  OutputSignals=I
  Bus Selector17 : BusSelector  OutputSignals=valid
  Bus Selector{18..25,27..34} (16 alike) : BusSelector  OutputSignals=Q
  Bus Selector26 : BusSelector  OutputSignals=valid
  Bus Selector35 : BusSelector  OutputSignals=ch
  Bus Selector36 : BusSelector  OutputSignals=ch
  DAC subSum : CryoDetLibCMB/DAC subSum
  DAC subSum1 : CryoDetLibCMB/DAC subSum
  In17 : InportShadow
  In18 : InportShadow  Port=2
  In19 : InportShadow  Port=3
  In20 : InportShadow  Port=4
  In21 : InportShadow  Port=5
  In22 : InportShadow  Port=6
  In23 : InportShadow  Port=7
  In24 : InportShadow  Port=8
  In25 : InportShadow  Port=9
  In26 : InportShadow  Port=10
  In27 : InportShadow  Port=11
  In28 : InportShadow  Port=12
  In29 : InportShadow  Port=13
  In30 : InportShadow  Port=14
  In31 : InportShadow  Port=15
  In32 : InportShadow  Port=16
  valid : Outport
  Q : Outport  Port=2
  I : Outport  Port=3
  ch : Outport  Port=4
  wires:
  DAC subSum/1 -> valid/1
  DAC subSum/2 -> I/1
  DAC subSum/3 -> ch/1
  DAC subSum1/2 -> Q/1
  Bus Selector36/1 -> DAC subSum1/18  "<ch>"
  Bus Selector35/1 -> DAC subSum/18  "<ch>"
  In1/1 -> Bus Selector17/1, Bus Selector35/1, Bus Selector2/1
  In2/1 -> Bus Selector1/1
  In3/1 -> Bus Selector3/1
  In4/1 -> Bus Selector4/1
  In5/1 -> Bus Selector6/1
  In6/1 -> Bus Selector5/1
  In7/1 -> Bus Selector7/1
  In8/1 -> Bus Selector8/1
  In9/1 -> Bus Selector10/1
  In10/1 -> Bus Selector9/1
  In11/1 -> Bus Selector11/1
  In12/1 -> Bus Selector12/1
  In13/1 -> Bus Selector13/1
  In14/1 -> Bus Selector16/1
  In15/1 -> Bus Selector14/1
  In16/1 -> Bus Selector15/1
  In17/1 -> Bus Selector36/1, Bus Selector26/1, Bus Selector27/1
  In18/1 -> Bus Selector18/1
  In19/1 -> Bus Selector28/1
  In20/1 -> Bus Selector29/1
  In21/1 -> Bus Selector31/1
  In22/1 -> Bus Selector19/1
  In23/1 -> Bus Selector20/1
  In24/1 -> Bus Selector21/1
  In25/1 -> Bus Selector22/1
  In26/1 -> Bus Selector23/1
  In27/1 -> Bus Selector24/1
  In28/1 -> Bus Selector25/1
  In29/1 -> Bus Selector30/1
  In30/1 -> Bus Selector32/1
  In31/1 -> Bus Selector33/1
  In32/1 -> Bus Selector34/1
  Bus Selector13/1 -> DAC subSum/14  "<I>"
  Bus Selector14/1 -> DAC subSum/16  "<I>"
  Bus Selector8/1 -> DAC subSum/9  "<I>"
  Bus Selector6/1 -> DAC subSum/6  "<I>"
  Bus Selector2/1 -> DAC subSum/2  "<I>"
  Bus Selector1/1 -> DAC subSum/3  "<I>"
  Bus Selector17/1 -> DAC subSum/1  "<valid>"
  Bus Selector15/1 -> DAC subSum/17  "<I>"
  Bus Selector10/1 -> DAC subSum/10  "<I>"
  Bus Selector11/1 -> DAC subSum/12  "<I>"
  Bus Selector12/1 -> DAC subSum/13  "<I>"
  Bus Selector16/1 -> DAC subSum/15  "<I>"
  Bus Selector3/1 -> DAC subSum/4  "<I>"
  Bus Selector7/1 -> DAC subSum/8  "<I>"
  Bus Selector4/1 -> DAC subSum/5  "<I>"
  Bus Selector9/1 -> DAC subSum/11  "<I>"
  Bus Selector5/1 -> DAC subSum/7  "<I>"
  Bus Selector23/1 -> DAC subSum1/11  "<Q>"
  Bus Selector18/1 -> DAC subSum1/3  "<Q>"
  Bus Selector32/1 -> DAC subSum1/15  "<Q>"
  Bus Selector25/1 -> DAC subSum1/13  "<Q>"
  Bus Selector31/1 -> DAC subSum1/6  "<Q>"
  Bus Selector33/1 -> DAC subSum1/16  "<Q>"
  Bus Selector21/1 -> DAC subSum1/9  "<Q>"
  Bus Selector19/1 -> DAC subSum1/7  "<Q>"
  Bus Selector29/1 -> DAC subSum1/5  "<Q>"
  Bus Selector20/1 -> DAC subSum1/8  "<Q>"
  Bus Selector28/1 -> DAC subSum1/4  "<Q>"
  Bus Selector27/1 -> DAC subSum1/2  "<Q>"
  Bus Selector34/1 -> DAC subSum1/17  "<Q>"
  Bus Selector30/1 -> DAC subSum1/14  "<Q>"
  Bus Selector22/1 -> DAC subSum1/10  "<Q>"
  Bus Selector24/1 -> DAC subSum1/12  "<Q>"
  Bus Selector26/1 -> DAC subSum1/1  "<valid>"
